simulink model "BLDC_speedcontrol_PWM"  (R2018a)
settings: Solver=ode45  StartTime=0.0  StopTime=2  FixedStep=Ts  MaxStep=.000001  RelTol=1e-3  EnableMultiTasking=on
InitFcn:
  | Power = 425;
  | 
  | R=.64;
  | L=1e-3;
  | J=.142e-3;
  | B=0;
  | Km=1.194;
  | Vdc=60;
  | 
  | Ts=1e-6;
  | P=16;
undefined symbols (not defined in the file): Ke, sigbuilder_block
libraries: powerlib x12, simulink x12, powerlib_meascontrol x8, dspsigops x4
settings Model: Creator=TELE  LastModifiedBy=TELE
settings SolverCC: ZeroCrossAlgorithm=Adaptive
settings DataIOCC: LimitDataPoints=on  SaveFormat=Array
settings OptimizationCC: LifeSpan=inf
settings DebuggingCC: UnderspecifiedInitializationDetection=Classic  MergeDetectMultiDrivingBlocksExec=none  MaxConsecutiveZCsMsg=none  SolverPrmCheckMsg=warning  StateNameClashWarn=warning  SFUnexpectedBacktrackingDiag=warning  SFNoUnconditionalDefaultTransitionDiag=warning  SFExecutionAtInitializationDiag=none
settings HardwareCC: ProdBitPerPointer=32  ProdBitPerSizeT=32  ProdBitPerPtrDiffT=32  ProdLargestAtomicFloat=None  ProdIntDivRoundTo=Undefined  ProdEndianess=Unspecified  ProdWordSize=32  ProdHWDeviceType=32-bit Generic
settings ModelReferenceCC: PropagateSignalLabelsOutOfModel=off
settings CodeAppCC: StateflowObjectComments=on
settings GRTTargetCC: TargetLangStandard=C89/C90 (ANSI)  GeneratePreprocessorConditionals=Disable all
settings ConfigComp: CovMetricSettings=dw  CovHtmlReporting=on  CovSaveCumulativeToWorkspaceVar=on  CovSaveSingleToWorkspaceVar=on  CovExternalEMLEnable=off
settings SimscapeCC: SimscapeNormalizeSystem=off

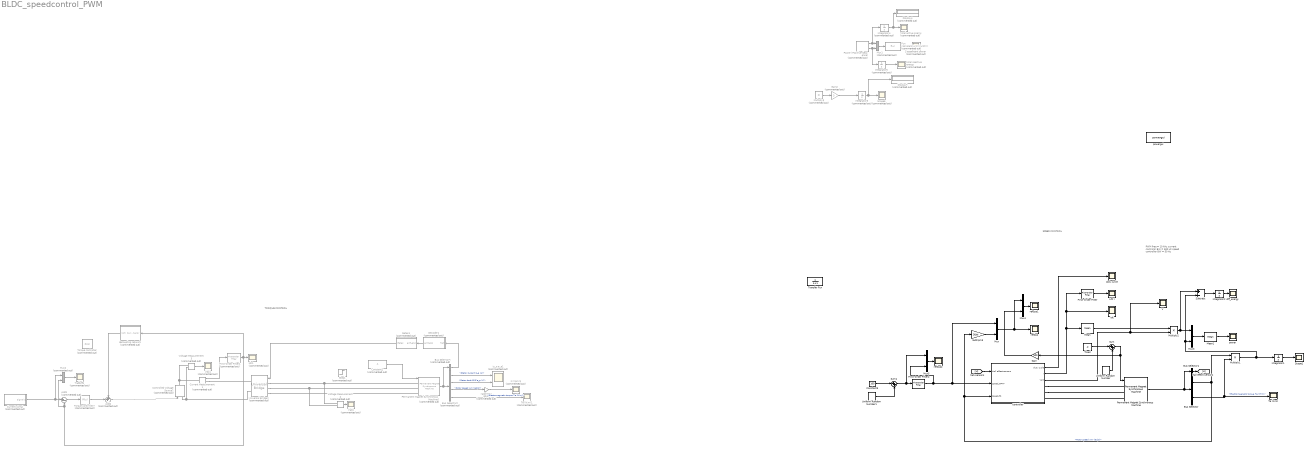
== system BLDC_speedcontrol_PWM ==
  note: SPEED CONTROL
  note: TORQUE CONTROL
  note: PWM freq = 10 kHz
      | current controler BW = 500 Hz
      | speed controller BW = 50 Hz
  Add1 : Sum  Commented=on  Inputs=|+-
  Add2 : Sum  Commented=on  Inputs=++|
  Bus Selector : BusSelector  OutputSignals=Rotor speed wm (rad/s),Electromagnetic torque Te (N*m)
  Bus Selector1 : BusSelector  OutputSignals=Hall effect signal h_a,Hall effect signal h_b,Hall effect signal h_c  OutputAsBus=on
  Bus Selector2 : BusSelector  Commented=on  OutputSignals=Stator current is_a (A),Stator back EMF e_a (V),Rotor speed wm (rad/s),Electromagnetic torque Te (N*m)
  Bus Selector3 : BusSelector  Commented=on  OutputSignals=Hall effect signal h_a,Hall effect signal h_b,Hall effect signal h_c  OutputAsBus=on
  Constant2 : Constant  Commented=on  Value=.1
  Constant3 : Constant  Value=100
  Controlled Voltage Source2 : powerlib/Electrical Sources/Controlled Voltage Source  Commented=on  Initialize=on  Source_Type=AC  Amplitude=500  Phase=0  Frequency=0  Measurements=None
  Current signal : Subsystem  Tag=STV Subsys  Commented=on  LoadFcn=sigbuilder_block('load');  StartFcn=sigbuilder_block('start');  StopFcn=sigbuilder_block('stop');  ClipboardFcn=sigbuilder_block('clipboard');  mask(Sigbuilder block){tuvar=[0:10]}
      mask help: Simulink:masks:SigbuilderBlock_MD
      mask init:
      | if ~strcmp(get_param(bdroot(gcbh),'SimulationStatus'),'stopped') tuvar = sigbuilder_block('maskInit'); end
      settings: CopyFcn=sigbuilder_block('copy');  DeleteFcn=sigbuilder_block('delete');  ModelCloseFcn=sigbuilder_block('modelClose');  PreSaveFcn=sigbuilder_block('preSave');  PauseFcn=sigbuilder_block('pause');  ContinueFcn=sigbuilder_block('continue');  NameChangeFcn=sigbuilder_block('namechange');  OpenFcn=sigbuilder_block('open',[437.25 180 550.5 395.25 ]);  CloseFcn=sigbuilder_block('close');
      mask Display: plot(0, 0, 100, 100,[2, 2, 32, 32, 2], [68, 8, 8, 68, 68],[32, 2], [38, 38], [32, 19, 2],[53, 60, 44], [32, 17, 17, 2],[16, 16, 31, 31]);txt = getActiveGroup(gcbh);text(2, 100, txt,'verticalAlignment', 'top');
  Current Measurement1 : powerlib/Measurements/Current Measurement  Commented=on  PhasorSimulation=off  OutputType=Complex  PSBequivalent=0
  Decoder1 : Subsystem  Commented=on
  Display3 : Display  Commented=on
  Display4 : Display  Commented=on
  Fcn : Fcn  Commented=on  Expr=cos(atan((u(1))/(u(2))))
  First-Order Filter : powerlib_meascontrol/Filters/First-Order Filter  FilterType=Lowpass  Tc=1e-3  Ts=0  Initialize=on  Vac_Init=[0, 0, 0]  Vdc_Init=0  PlotResponse=off  FreqRange="[0,  200,  1]"
      settings: SourceProductName=Simscape Power Systems
  First-Order Filter1 : powerlib_meascontrol/Filters/First-Order Filter  Commented=on  FilterType=Lowpass  Tc=10e-3  Ts=0  Initialize=on  Vac_Init=[0, 0, 60]  Vdc_Init=0  PlotResponse=off  FreqRange="[0,  200,  1]"
      settings: SourceProductName=Simscape Power Systems
  First-Order Filter2 : powerlib_meascontrol/Filters/First-Order Filter  FilterType=Lowpass  Tc=1/50  Ts=0  Initialize=on  Vac_Init=[0, 0, 0]  Vdc_Init=0  PlotResponse=off  FreqRange="[0,  200,  1]"
      settings: SourceProductName=Simscape Power Systems
  Gain : Gain  Gain=100
  Gain2 : Gain  Commented=on  Gain=3
  Gates1 : Subsystem  Commented=on
  "Idc " : Scope
  Idc1 : Scope  Commented=on
  Integrator1 : Integrator
  Integrator2 : Integrator
  Integrator3 : Integrator  Commented=on
  Integrator4 : Integrator  Commented=on
  Integrator5 : Integrator  Commented=on
  LPF I : Scope
  Mean : powerlib_meascontrol/Measurements/Mean  Freq=60  Vinit=0  Ts=0
  Mean1 : powerlib_meascontrol/Measurements/Mean  Freq=60  Vinit=0  Ts=0
  Multiply1 : Product
  Multiply2 : Product
  Multiply3 : Product  Commented=on
  Mux{,3..5} (4 alike) : Mux  Inputs=2
  Mux1 : Mux  Commented=on  Inputs=2
  Mux2 : Mux  Commented=on  Inputs=2
  N (rpm)1 : Scope  Commented=on
  Permanent Magnet Synchronous Machine : powerlib/Machines/Permanent Magnet Synchronous Machine  NbPhases=3  FluxDistribution=Trapezoidal  RotorType=Round  MechanicalLoad=Torque Tm  PresetModel=No  ShowDetailedParameters=on  MeasurementBus=off  Resistance=R  Inductance=L  dqInductances=[8.5e-3,8.5e-3]  La=L  MachineConstant=Torque Constant (N.m / A_peak)  Flux=0.037313  VoltageCst=125.0354  TorqueCst=Km  Flat=120  Mechanical=[J B P 0]  PolePairs=4  InitialConditions=[0,0, 0,0]  InitialConditions5ph=[0 0 0 0 0 0]  TsPowergui=0  TsBlock=-1  RefAngle=90 degrees behind phase A axis (modified Park)
      settings: SourceProductName=Simscape Power Systems
  Permanent Magnet Synchronous Machine1 : powerlib/Machines/Permanent Magnet Synchronous Machine  Commented=on  NbPhases=3  FluxDistribution=Trapezoidal  RotorType=Round  MechanicalLoad=Torque Tm  PresetModel=No  ShowDetailedParameters=on  MeasurementBus=off  Resistance=R  Inductance=L  dqInductances=[8.5e-3, 8.5e-3]  La=0.000835  MachineConstant=Torque Constant (N.m / A_peak)  Flux=0.00425  VoltageCst=7.1209  TorqueCst=Kt  Flat=120  Mechanical=[ J, B 8]  PolePairs=8  InitialConditions=[0,0, 0,0]  InitialConditions5ph=[0 0 0 0 0 0]  TsPowergui=0  TsBlock=-1  RefAngle=90 degrees behind phase A axis (modified Park)
      settings: SourceProductName=Simscape Power Systems
  Power (Positive-Sequence) : powerlib_meascontrol/Measurements/Power (Positive-Sequence)  Commented=on  Freq=60  Vinit=[0, 0]  Iinit=[0, 0]  Ts=0
      settings: SourceProductName=Simscape Power Systems  SourceProductBaseCode=PS
  S appereant power : Scope  Commented=on
  Scope1 : Scope
  Scope6 : Scope  Commented=on
  Step1 : Step  Commented=on  After=.1  SampleTime=0
  Subtract : Sum  Inputs=+-
  Sum : Sum  Inputs=|++
  Sum1 : Sum  Inputs=|++
  Te (N.m) : Scope
  Te (N.m)1 : Scope  Commented=on
  Tload : Constant  Value=.2
  Torque controller : simulink/Continuous/PID Controller  Commented=on  Controller=PI  TimeDomain=Continuous-time  SampleTime=-1  IntegratorMethod=Forward Euler  FilterMethod=Forward Euler  Form=Parallel  UseFilter=on  ControllerParametersSource=internal  P=2.12871841993777  I=6083.3305788616*.5  D=-0.000138058001454029  N=230.258625302705  InitialConditionSource=internal  InitialConditionForIntegrator=0  InitialConditionForFilter=0  ExternalReset=none  LimitOutput=off  UpperSaturationLimit=inf  LowerSaturationLimit=-inf  LinearizeAsGain=on  AntiWindupMode=none  Kb=1  TrackingMode=off  Kt=1  PParamMin=[]  PParamMax=[]  IParamMin=[]  IParamMax=[]  DParamMin=[]  DParamMax=[]  NParamMin=[]  NParamMax=[]  KbParamMin=[]  KbParamMax=[]  KtParamMin=[]  KtParamMax=[]  POutMin=[]  POutMax=[]  IOutMin=[]  IOutMax=[]  DOutMin=[]  DOutMax=[]  NOutMin=[]  NOutMax=[]  KbOutMin=[]  KbOutMax=[]  KtOutMin=[]  KtOutMax=[]  IntegratorOutMin=[]  IntegratorOutMax=[]  FilterOutMin=[]  FilterOutMax=[]  SumOutMin=[]  SumOutMax=[]  SumI1OutMin=[]  SumI1OutMax=[]  SumI2OutMin=[]  SumI2OutMax=[]  SumI3OutMin=[]  SumI3OutMax=[]  SumDOutMin=[]  SumDOutMax=[]  SaturationOutMin=[]  SaturationOutMax=[]  IntegratorContinuousStateAttributes=''  IntegratorStateMustResolveToSignalObject=off  IntegratorRTWStateStorageClass=Auto  FilterContinuousStateAttributes=''  FilterStateMustResolveToSignalObject=off  FilterRTWStateStorageClass=Auto  DifferentiatorICPrevScaledInput=0  DifferentiatorOutMin=[]  DifferentiatorOutMax=[]  FilterDiffOutCoefMin=[]  FilterDiffOutCoefMax=[]  SumDenOutMin=[]  SumDenOutMax=[]  SumNumOutMin=[]  SumNumOutMax=[]  ReciprocalOutMin=[]  ReciprocalOutMax=[]  DivideOutMin=[]  DivideOutMax=[]  TunerSelectOption=Transfer Function Based (PID Tuner App)
  Torque controller2 : simulink/Continuous/PID Controller  Commented=on  Controller=PI  TimeDomain=Continuous-time  SampleTime=-1  IntegratorMethod=Forward Euler  FilterMethod=Forward Euler  Form=Parallel  UseFilter=on  ControllerParametersSource=internal  P=7.77723774722096  I=2722.31111979485  D=-0.000138058001454029  N=230.258625302705  InitialConditionSource=internal  InitialConditionForIntegrator=0  InitialConditionForFilter=0  ExternalReset=none  LimitOutput=off  UpperSaturationLimit=inf  LowerSaturationLimit=-inf  LinearizeAsGain=on  AntiWindupMode=none  Kb=1  TrackingMode=off  Kt=1  PParamMin=[]  PParamMax=[]  IParamMin=[]  IParamMax=[]  DParamMin=[]  DParamMax=[]  NParamMin=[]  NParamMax=[]  KbParamMin=[]  KbParamMax=[]  KtParamMin=[]  KtParamMax=[]  POutMin=[]  POutMax=[]  IOutMin=[]  IOutMax=[]  DOutMin=[]  DOutMax=[]  NOutMin=[]  NOutMax=[]  KbOutMin=[]  KbOutMax=[]  KtOutMin=[]  KtOutMax=[]  IntegratorOutMin=[]  IntegratorOutMax=[]  FilterOutMin=[]  FilterOutMax=[]  SumOutMin=[]  SumOutMax=[]  SumI1OutMin=[]  SumI1OutMax=[]  SumI2OutMin=[]  SumI2OutMax=[]  SumI3OutMin=[]  SumI3OutMax=[]  SumDOutMin=[]  SumDOutMax=[]  SaturationOutMin=[]  SaturationOutMax=[]  IntegratorContinuousStateAttributes=''  IntegratorStateMustResolveToSignalObject=off  IntegratorRTWStateStorageClass=Auto  FilterContinuousStateAttributes=''  FilterStateMustResolveToSignalObject=off  FilterRTWStateStorageClass=Auto  DifferentiatorICPrevScaledInput=0  DifferentiatorOutMin=[]  DifferentiatorOutMax=[]  FilterDiffOutCoefMin=[]  FilterDiffOutCoefMax=[]  SumDenOutMin=[]  SumDenOutMax=[]  SumNumOutMin=[]  SumNumOutMax=[]  ReciprocalOutMin=[]  ReciprocalOutMax=[]  DivideOutMin=[]  DivideOutMax=[]  TunerSelectOption=Transfer Function Based (PID Tuner App)
  Transfer Fcn : TransferFcn  Denominator=[1 1]
  Tref&Tfb : Scope  Commented=on
  Uniform Random Number : UniformRandomNumber  Minimum=0  SampleTime=.1
  Uniform Random Number1 : UniformRandomNumber  Minimum=0  Maximum=200  SampleTime=1/100
  Universal Bridge1 : powerlib/Power Electronics/Universal Bridge  Commented=on  Arms=3  SnubberResistance=5000  SnubberCapacitance=1e-6  Device=MOSFET / Diodes  Ron=1e-3  Lon=0  ForwardVoltages="[  0  0  ]"  ForwardVoltage=0  GTOparameters=[ 10e-6 , 20e-6 ]  IGBTparameters=[ 1e-6 , 2e-6 ]  Measurements=None  Measurements_2=None  converterType=Rectifier
  V : Scope
  Vab1 : Scope  Commented=on
  Vdc1 : Scope  Commented=on
  Voltage Measurement2 : powerlib/Measurements/Voltage Measurement  Commented=on  PhasorSimulation=off  OutputType=Complex  PSBequivalent=0
  Voltage Measurement3 : powerlib/Measurements/Voltage Measurement  Commented=on  PhasorSimulation=off  OutputType=Complex  PSBequivalent=0
  controller : Subsystem
  decoupling network : Subsystem  Commented=on
  diff_energy : Scope
  duty cycle : Scope
  is_a e_a1 : Scope  Commented=on  NumInputPorts=2
  power : Scope
  powergui : powerlib/powergui  Priority=2  SimulationMode=Continuous  SampleTime=Ts  frequency=60  Iterations=50  frequencyindice=0  Pbase=100e6  ErrMax=1e-4  UnitsV=kV  UnitsW=MW  buscounter=0  FunctionMessages=off  echomessages=off  EnableUseOfTLC=off  CurrentSourceSwitches=off  DisableSnubberDevices=off  DisableRonSwitches=off  DisableVfSwitches=off  DisplayEquations=off  SolverType=Tustin  Interpol=off  ExternalGateDelay=off  methode=off  Ts=0  x0status=blocks  SPID=off  SwTol=0  HookPort=off  RestoreLinks=warning  ResistiveCurrentMeasurement=off  Frange=[0:2:500]  Ylog=off  Xlog=on  ShowGrid=off  save=off  variable=ZData  structure=0  ZoomFFT=on  StartTime=0.0  cycles=1  DisplayStyle=1  fundamental=60  FreqAxis=off  MaxFrequency=1000  frequencyindicesteady=1  RmsSteady=1  display=off
  rad2rpm1 : Gain  Commented=on  Gain=30/pi
  rad2rpm3 : Gain  Gain=30/pi
  ref&sp : Scope
  ref&sp1 : Scope
  ref&sp2 : Scope
  total active energy : Scope  Commented=on
  total reactive energy : Scope  Commented=on
  wires:
  Permanent Magnet Synchronous Machine/1 -> Bus Selector1/1, Bus Selector/1
  Bus Selector1/1 -> [H]
  Bus Selector/1 -> Multiply1/1, rad2rpm3/1, controller/3(speed_fb)  "<Rotor speed wm (rad/s)>"
  Bus Selector/2 -> Multiply1/2, Te (N.m)/1  "<Electromagnetic torque Te (N*m)>"
  Gates1/1(Gates) -> Universal Bridge1/1
  Decoder1/1(emf_abc) -> Gates1/1("emf_abc ")
  rad2rpm1/1 -> N (rpm)1/1
  Voltage Measurement2/1 -> Vab1/1
  Voltage Measurement3/1 -> Vdc1/1
  Bus Selector2/1 -> is_a e_a1/1  "<Stator current is_a (A)>"
  Permanent Magnet Synchronous Machine1/1 -> Bus Selector2/1, Bus Selector3/1
  Bus Selector3/1 -> Decoder1/1("Hall ")
  Bus Selector2/2 -> is_a e_a1/2  "<Stator back EMF e_a (V)>"
  Bus Selector2/3 -> rad2rpm1/1  "<Rotor speed wm (rad/s)>"
  Bus Selector2/4 -> Te (N.m)1/1  "<Electromagnetic torque Te (N*m)>"
  Current Measurement1/1 -> First-Order Filter1/1
  Add1/1 -> Torque controller2/1
  Mux2/1 -> Tref&Tfb/1
  First-Order Filter1/1 -> decoupling network/1(Current error), Mux2/2, Add1/2, Idc1/1
  Current signal/1(Signal 1) -> Mux2/1, Add1/1
  Constant2/1 -> Permanent Magnet Synchronous Machine1/1
  Torque controller2/1 -> Add2/2
  Add2/1 -> Controlled Voltage Source2/1
  decoupling network/1(Volt) -> Add2/1
  [H] -> controller/1(Hall effect sensors)
  controller/1(duty cycle) -> duty cycle/1
  Integrator1/1 -> Scope1/1
  Mux/1 -> ref&sp/1, Mux4/1
  rad2rpm3/1 -> Mux/2
  Gain2/1 -> Integrator3/1
  Integrator3/1 -> Display3/1, Scope6/1
  Multiply3/1 -> Gain2/1
  Integrator5/1 -> total reactive energy/1
  Power (Positive-Sequence)/1 -> Integrator4/1, Mux1/1
  Mux1/1 -> Fcn/1
  ? -> Power (Positive-Sequence)/2
  Integrator4/1 -> Display4/1, total active energy/1
  Fcn/1 -> S appereant power/1
  Power (Positive-Sequence)/2 -> Integrator5/1, Mux1/2
  ? -> Power (Positive-Sequence)/1
  Tload/1 -> Sum/1
  controller/2(I) -> First-Order Filter/1, "Idc "/1, Mean/1
  First-Order Filter/1 -> LPF I/1
  Subtract/1 -> Integrator2/1
  Mean/1 -> Multiply2/1
  controller/3(Volt) -> V/1, Multiply2/2
  Mux3/1 -> Mean1/1
  Multiply2/1 -> Subtract/1, Mux3/1
  Multiply1/1 -> Subtract/2, Mux3/2, Integrator1/1
  Integrator2/1 -> diff_energy/1
  Uniform Random Number/1 -> Sum/2
  Mux4/1 -> ref&sp1/1
  Sum/1 -> Permanent Magnet Synchronous Machine/1, Gain/1
  Gain/1 -> Mux4/2
  Mean1/1 -> power/1
  Sum1/1 -> First-Order Filter2/1, Mux5/1
  Mux5/1 -> ref&sp2/1
  Constant3/1 -> Sum1/1
  Uniform Random Number1/1 -> Sum1/2
  First-Order Filter2/1 -> Mux5/2, Mux/1, controller/2(speed_RPM*)
  connections:
  Universal Bridge1/LConn1 -- Voltage Measurement2/LConn1 -- Permanent Magnet Synchronous Machine1/LConn1
  Universal Bridge1/LConn2 -- Voltage Measurement2/LConn2 -- Permanent Magnet Synchronous Machine1/LConn2
  Controlled Voltage Source2/RConn1 -- Current Measurement1/LConn1 -- Voltage Measurement3/LConn1
  Controlled Voltage Source2/LConn1 -- Voltage Measurement3/LConn2 -- Universal Bridge1/RConn2
  Universal Bridge1/LConn3 -- Permanent Magnet Synchronous Machine1/LConn3
  Current Measurement1/RConn1 -- Universal Bridge1/RConn1
  Permanent Magnet Synchronous Machine/LConn3 -- controller/RConn3
  controller/RConn2 -- Permanent Magnet Synchronous Machine/LConn2
  controller/RConn1 -- Permanent Magnet Synchronous Machine/LConn1

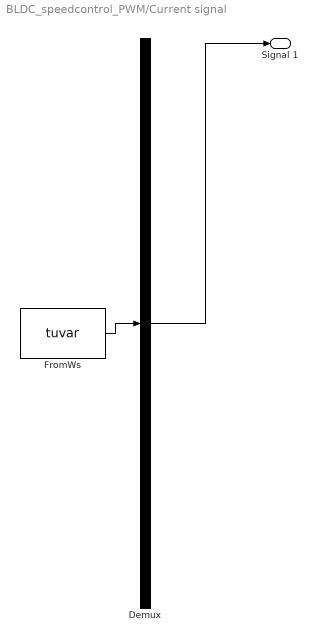
== system BLDC_speedcontrol_PWM/Current signal ==
  Demux : Demux  Tag=STV Demux  Outputs=1
  FromWs : FromWorkspace  Tag=STV FromWs  VariableName=tuvar  SampleTime=0
      SigBuilderData=|
      | common.afterFinalStr = 'Extrapolate'
      | common.sampleTime = 0
      | dataSet.timeRange = [0 10]
      | dataSet.name = 'Group 1'
      | sbobj.Groups.Name = 'Group 1'
      | sbobj.Groups.Signals.Name = 'Signal 1'
      | sbobj.Groups.Signals.XData = [0 0.22 0.22 2 2 10]
      | sbobj.Groups.Signals.YData = [0 0 2 2 0 0]
  Signal 1 : Outport  Tag=STV Outport
  wires:
  FromWs/1 -> Demux/1
  Demux/1 -> Signal 1/1

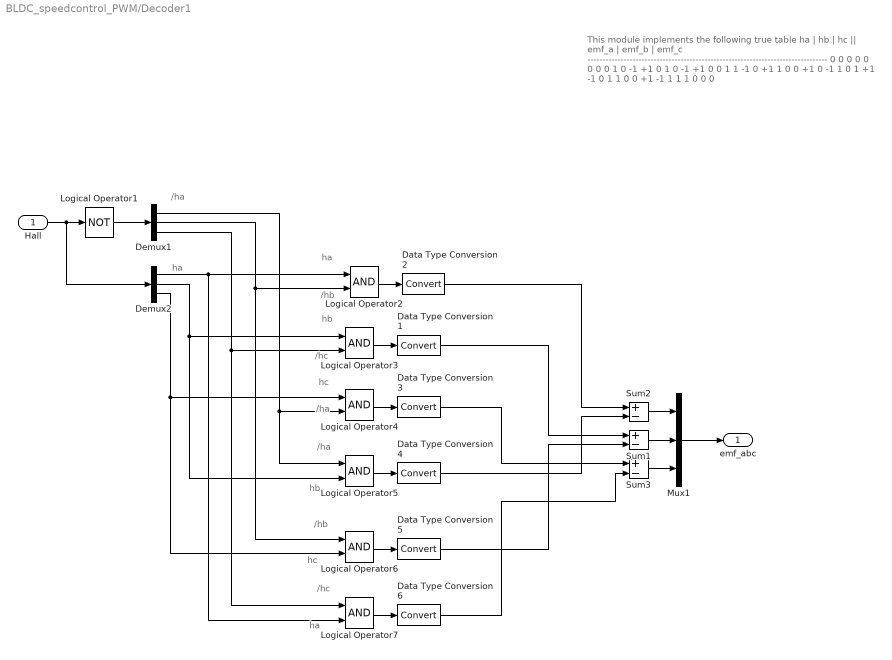
== system BLDC_speedcontrol_PWM/Decoder1 ==
  note: /ha
  note: ha
  note: ha
  note: /hb
  note: hb
  note: /hc
  note: hc
  note: /ha
  note: /ha
  note: hb
  note: /hb
  note: hc
  note: /hc
  note: ha
  note: This module implements the following true table
      |
      |    ha   |   hb   |   hc   ||   emf_a   |   emf_b   |   emf_c
      |     --------------------------------------------------------------------------------
      | 0          0         0          0               0               0
      | 0          0         1          0               -1              +1
      | 0          1         0          -1              +1                0
      | 0          1         1          -1               0               +1
      | 1          0         0         +1               0               -1
      | 1          0         1         +1              -1                0
      | 1          1         0          0              +1               -1
      | 1          1         1          0               0                0
  "Hall " : Inport
  Data Type Conversion{1..6} (6 alike) : DataTypeConversion
  Demux1 : Demux  Outputs=3
  Demux2 : Demux  Outputs=3
  Logical Operator1 : Logic  Operator=NOT  AllPortsSameDT=off  OutDataTypeStr=boolean
  Logical Operator{2..7} (6 alike) : Logic  AllPortsSameDT=off  OutDataTypeStr=boolean
  Mux1 : Mux  Inputs=3
  Sum1 : Sum  Inputs=+-  OutDataTypeStr=double
  Sum2 : Sum  Inputs=+-  OutDataTypeStr=double
  Sum3 : Sum  Inputs=+-  OutDataTypeStr=double
  emf_abc : Outport
  wires:
  "Hall "/1 -> Logical Operator1/1, Demux2/1
  Logical Operator1/1 -> Demux1/1
  Demux2/3 -> Logical Operator4/1, Logical Operator6/2
  Demux2/2 -> Logical Operator3/1, Logical Operator5/2
  Demux2/1 -> Logical Operator2/1, Logical Operator7/2
  Demux1/3 -> Logical Operator3/2, Logical Operator7/1
  Demux1/2 -> Logical Operator2/2, Logical Operator6/1
  Demux1/1 -> Logical Operator4/2, Logical Operator5/1
  Logical Operator2/1 -> Data Type Conversion2/1
  Sum2/1 -> Mux1/1
  Sum1/1 -> Mux1/2
  Sum3/1 -> Mux1/3
  Mux1/1 -> emf_abc/1
  Logical Operator3/1 -> Data Type Conversion1/1
  Logical Operator4/1 -> Data Type Conversion3/1
  Logical Operator5/1 -> Data Type Conversion4/1
  Logical Operator6/1 -> Data Type Conversion5/1
  Logical Operator7/1 -> Data Type Conversion6/1
  Data Type Conversion2/1 -> Sum2/1
  Data Type Conversion4/1 -> Sum2/2
  Data Type Conversion1/1 -> Sum1/1
  Data Type Conversion5/1 -> Sum1/2
  Data Type Conversion3/1 -> Sum3/1
  Data Type Conversion6/1 -> Sum3/2

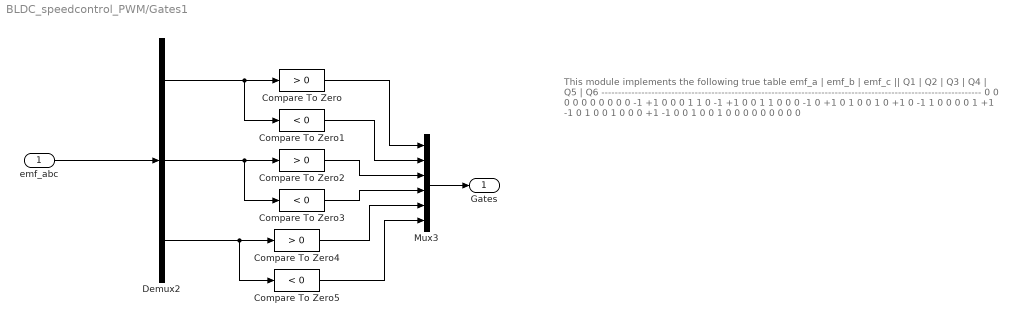
== system BLDC_speedcontrol_PWM/Gates1 ==
  note: This module implements the following true table
      |
      |    emf_a   |   emf_b   |   emf_c   ||   Q1   |   Q2   |   Q3   |   Q4   |   Q5   |   Q6
      |     ------------------------------------------------------------------------------------------------------------------
      |       0              0                0            0          0          0           0        0        0
      |       0               -1              +1          0          0          0           1        1        0
      |     -1              +1                0          0          1          1           0        0        0
      |     -1               0               +1          0          1         0           0        1        0
      |    +1               0                -1          1          0          0           0        0        1
      |    +1              -1                0           1          0          0           1        0        0
      |      0              +1               -1           0          0          1           0        0        1
      |     0              0                0             0          0          0           0        0        0
  "emf_abc " : Inport
  Compare To Zero : simulink/Logic and Bit Operations/Compare To Zero  relop=>  OutDataTypeStr=boolean  ZeroCross=off
  Compare To Zero1 : simulink/Logic and Bit Operations/Compare To Zero  relop=<  OutDataTypeStr=boolean  ZeroCross=off
  Compare To Zero2 : simulink/Logic and Bit Operations/Compare To Zero  relop=>  OutDataTypeStr=boolean  ZeroCross=off
  Compare To Zero3 : simulink/Logic and Bit Operations/Compare To Zero  relop=<  OutDataTypeStr=boolean  ZeroCross=off
  Compare To Zero4 : simulink/Logic and Bit Operations/Compare To Zero  relop=>  OutDataTypeStr=boolean  ZeroCross=off
  Compare To Zero5 : simulink/Logic and Bit Operations/Compare To Zero  relop=<  OutDataTypeStr=boolean  ZeroCross=off
  Demux2 : Demux  Outputs=3
  Mux3 : Mux  Inputs=6
  Gates : Outport
  wires:
  "emf_abc "/1 -> Demux2/1
  Mux3/1 -> Gates/1
  Demux2/1 -> Compare To Zero/1, Compare To Zero1/1
  Demux2/2 -> Compare To Zero2/1, Compare To Zero3/1
  Demux2/3 -> Compare To Zero4/1, Compare To Zero5/1
  Compare To Zero/1 -> Mux3/1
  Compare To Zero1/1 -> Mux3/2
  Compare To Zero2/1 -> Mux3/3
  Compare To Zero3/1 -> Mux3/4
  Compare To Zero4/1 -> Mux3/5
  Compare To Zero5/1 -> Mux3/6

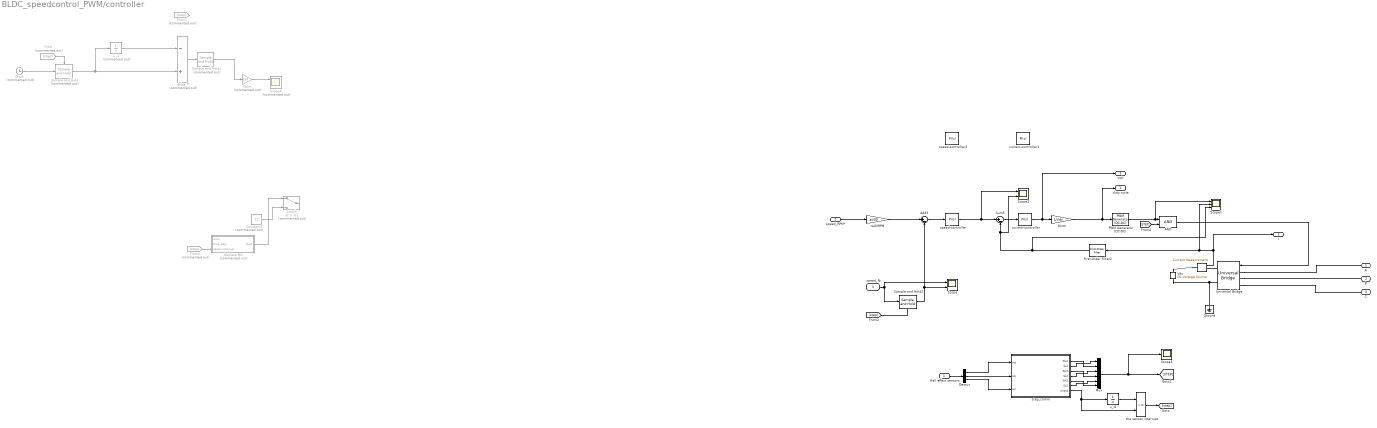
== system BLDC_speedcontrol_PWM/controller ==
  Hall effect sensors : Inport
  speed_RPM* : Inport  Port=2
  speed_fb : Inport  Port=3
  ' : powerlib/Measurements/Current Measurement  PhasorSimulation=off  OutputType=Complex  PSBequivalent=0
  AND : Logic  AllPortsSameDT=off  OutDataTypeStr=boolean
  Add3 : Sum  Inputs=|+-
  Clock : Clock  Commented=on
  Constant1 : Constant  Commented=on  Value=12
  Demux : Demux  Outputs=3
  First-Order Filter2 : powerlib_meascontrol/Filters/First-Order Filter  FilterType=Lowpass  Tc=1e-3  Ts=0  Initialize=on  Vac_Init=[0, 0, 0]  Vdc_Init=0  PlotResponse=off  FreqRange="[0,  200,  1]"
      settings: SourceProductName=Simscape Power Systems
  From : From  Commented=on  GotoTag=step
  From1 : From  Commented=on  GotoTag=step
  From3 : From  Commented=on  GotoTag=step
  Gain : Gain  Commented=on  Gain=1e3
  Ground : powerlib/Elements/Ground  LConnTagsString=a
  Mux : Mux  Inputs=6
  Norm : Gain  Gain=1/Vdc
  PWM Generator (DC-DC) : powerlib_meascontrol/Pulse & Signal Generators/PWM Generator (DC-DC)  Fsw=20e3  Ts=0
  Sample and Hold : dspsigops/Sample and Hold  Commented=on  trig=Rising edge  initCond=0  latchinput=off
  Sample and Hold1 : dspsigops/Sample and Hold  Commented=on  trig=Rising edge  initCond=0  latchinput=off
  Sample and Hold2 : dspsigops/Sample and Hold  trig=Rising edge  initCond=0  latchinput=off
  Scope : Scope  NumInputPorts=2
  Scope1 : Scope  NumInputPorts=3
  Scope2 : Scope  NumInputPorts=2
  Scope4 : Scope  Commented=on  NumInputPorts=2
  Scope5 : Scope
  Sum5 : Sum  Inputs=|+-
  Switch : Switch  Commented=on  Criteria=u2 > Threshold  Threshold=.01
  Universal Bridge : powerlib/Power Electronics/Universal Bridge  Arms=3  SnubberResistance=5000  SnubberCapacitance=1e-6  Device=MOSFET / Diodes  Ron=1e-3  Lon=0  ForwardVoltages="[  0  0  ]"  ForwardVoltage=0  GTOparameters=[ 10e-6 , 20e-6 ]  IGBTparameters=[ 1e-6 , 2e-6 ]  Measurements=None  Measurements_2=None  converterType=Rectifier
  Vdc : powerlib/Electrical Sources/DC Voltage Source  Amplitude=Vdc  Measurements=None
  current-controller : simulink/Continuous/PID Controller  Controller=PI  TimeDomain=Continuous-time  SampleTime=-1  IntegratorMethod=Forward Euler  FilterMethod=Forward Euler  Form=Parallel  UseFilter=on  ControllerParametersSource=internal  P=.01  I=479.896371550439  D=-0.000138058001454029  N=230.258625302705  InitialConditionSource=internal  InitialConditionForIntegrator=0  InitialConditionForFilter=0  ExternalReset=none  LimitOutput=on  UpperSaturationLimit=Vdc  LowerSaturationLimit=0  LinearizeAsGain=on  AntiWindupMode=clamping  Kb=1  TrackingMode=off  Kt=1  PParamMin=[]  PParamMax=[]  IParamMin=[]  IParamMax=[]  DParamMin=[]  DParamMax=[]  NParamMin=[]  NParamMax=[]  KbParamMin=[]  KbParamMax=[]  KtParamMin=[]  KtParamMax=[]  POutMin=[]  POutMax=[]  IOutMin=[]  IOutMax=[]  DOutMin=[]  DOutMax=[]  NOutMin=[]  NOutMax=[]  KbOutMin=[]  KbOutMax=[]  KtOutMin=[]  KtOutMax=[]  IntegratorOutMin=[]  IntegratorOutMax=[]  FilterOutMin=[]  FilterOutMax=[]  SumOutMin=[]  SumOutMax=[]  SumI1OutMin=[]  SumI1OutMax=[]  SumI2OutMin=[]  SumI2OutMax=[]  SumI3OutMin=[]  SumI3OutMax=[]  SumDOutMin=[]  SumDOutMax=[]  SaturationOutMin=[]  SaturationOutMax=[]  IntegratorContinuousStateAttributes=''  IntegratorStateMustResolveToSignalObject=off  IntegratorRTWStateStorageClass=Auto  FilterContinuousStateAttributes=''  FilterStateMustResolveToSignalObject=off  FilterRTWStateStorageClass=Auto  DifferentiatorICPrevScaledInput=0  DifferentiatorOutMin=[]  DifferentiatorOutMax=[]  FilterDiffOutCoefMin=[]  FilterDiffOutCoefMax=[]  SumDenOutMin=[]  SumDenOutMax=[]  SumNumOutMin=[]  SumNumOutMax=[]  ReciprocalOutMin=[]  ReciprocalOutMax=[]  DivideOutMin=[]  DivideOutMax=[]  TunerSelectOption=Transfer Function Based (PID Tuner App)
  current-controller1 : simulink/Continuous/PID Controller  Controller=PI  TimeDomain=Discrete-time  SampleTime=.0002  IntegratorMethod=Trapezoidal  FilterMethod=Forward Euler  Form=Parallel  UseFilter=on  ControllerParametersSource=internal  P=0.228414146935332  I=376.292717854929  D=-0.000138058001454029  N=230.258625302705  InitialConditionSource=internal  InitialConditionForIntegrator=0  InitialConditionForFilter=0  ExternalReset=none  LimitOutput=on  UpperSaturationLimit=Vdc  LowerSaturationLimit=0  LinearizeAsGain=on  AntiWindupMode=clamping  Kb=1  TrackingMode=off  Kt=1  PParamMin=[]  PParamMax=[]  IParamMin=[]  IParamMax=[]  DParamMin=[]  DParamMax=[]  NParamMin=[]  NParamMax=[]  KbParamMin=[]  KbParamMax=[]  KtParamMin=[]  KtParamMax=[]  POutMin=[]  POutMax=[]  IOutMin=[]  IOutMax=[]  DOutMin=[]  DOutMax=[]  NOutMin=[]  NOutMax=[]  KbOutMin=[]  KbOutMax=[]  KtOutMin=[]  KtOutMax=[]  IntegratorOutMin=[]  IntegratorOutMax=[]  FilterOutMin=[]  FilterOutMax=[]  SumOutMin=[]  SumOutMax=[]  SumI1OutMin=[]  SumI1OutMax=[]  SumI2OutMin=[]  SumI2OutMax=[]  SumI3OutMin=[]  SumI3OutMax=[]  SumDOutMin=[]  SumDOutMax=[]  SaturationOutMin=[]  SaturationOutMax=[]  IntegratorContinuousStateAttributes=''  IntegratorStateMustResolveToSignalObject=off  IntegratorRTWStateStorageClass=Auto  FilterContinuousStateAttributes=''  FilterStateMustResolveToSignalObject=off  FilterRTWStateStorageClass=Auto  DifferentiatorICPrevScaledInput=0  DifferentiatorOutMin=[]  DifferentiatorOutMax=[]  FilterDiffOutCoefMin=[]  FilterDiffOutCoefMax=[]  SumDenOutMin=[]  SumDenOutMax=[]  SumNumOutMin=[]  SumNumOutMax=[]  ReciprocalOutMin=[]  ReciprocalOutMax=[]  DivideOutMin=[]  DivideOutMax=[]  TunerSelectOption=Transfer Function Based (PID Tuner App)
  delta_T : Sum  Commented=on  Inputs=-+
  discrete PID : Subsystem  Commented=on
  rad2RPM : Gain  Gain=pi/30
  speed-controller : simulink/Continuous/PID Controller  Controller=PI  TimeDomain=Continuous-time  SampleTime=-1  IntegratorMethod=Forward Euler  FilterMethod=Forward Euler  Form=Parallel  UseFilter=on  ControllerParametersSource=internal  P=0.185814513304236  I=4.94881180882956  D=-0.000138058001454029  N=230.258625302705  InitialConditionSource=internal  InitialConditionForIntegrator=0  InitialConditionForFilter=0  ExternalReset=none  LimitOutput=on  UpperSaturationLimit=Vdc  LowerSaturationLimit=0  LinearizeAsGain=on  AntiWindupMode=clamping  Kb=1  TrackingMode=off  Kt=1  PParamMin=[]  PParamMax=[]  IParamMin=[]  IParamMax=[]  DParamMin=[]  DParamMax=[]  NParamMin=[]  NParamMax=[]  KbParamMin=[]  KbParamMax=[]  KtParamMin=[]  KtParamMax=[]  POutMin=[]  POutMax=[]  IOutMin=[]  IOutMax=[]  DOutMin=[]  DOutMax=[]  NOutMin=[]  NOutMax=[]  KbOutMin=[]  KbOutMax=[]  KtOutMin=[]  KtOutMax=[]  IntegratorOutMin=[]  IntegratorOutMax=[]  FilterOutMin=[]  FilterOutMax=[]  SumOutMin=[]  SumOutMax=[]  SumI1OutMin=[]  SumI1OutMax=[]  SumI2OutMin=[]  SumI2OutMax=[]  SumI3OutMin=[]  SumI3OutMax=[]  SumDOutMin=[]  SumDOutMax=[]  SaturationOutMin=[]  SaturationOutMax=[]  IntegratorContinuousStateAttributes=''  IntegratorStateMustResolveToSignalObject=off  IntegratorRTWStateStorageClass=Auto  FilterContinuousStateAttributes=''  FilterStateMustResolveToSignalObject=off  FilterRTWStateStorageClass=Auto  DifferentiatorICPrevScaledInput=0  DifferentiatorOutMin=[]  DifferentiatorOutMax=[]  FilterDiffOutCoefMin=[]  FilterDiffOutCoefMax=[]  SumDenOutMin=[]  SumDenOutMax=[]  SumNumOutMin=[]  SumNumOutMax=[]  ReciprocalOutMin=[]  ReciprocalOutMax=[]  DivideOutMin=[]  DivideOutMax=[]  TunerSelectOption=Transfer Function Based (PID Tuner App)
  speed-controller2 : simulink/Continuous/PID Controller  Controller=PI  TimeDomain=Discrete-time  SampleTime=.0002  IntegratorMethod=Trapezoidal  FilterMethod=Forward Euler  Form=Parallel  UseFilter=on  ControllerParametersSource=internal  P=0.127599674617565  I=1.78394081781165  D=-0.000138058001454029  N=230.258625302705  InitialConditionSource=internal  InitialConditionForIntegrator=0  InitialConditionForFilter=0  ExternalReset=none  LimitOutput=on  UpperSaturationLimit=Vdc  LowerSaturationLimit=0  LinearizeAsGain=on  AntiWindupMode=clamping  Kb=1  TrackingMode=off  Kt=1  PParamMin=[]  PParamMax=[]  IParamMin=[]  IParamMax=[]  DParamMin=[]  DParamMax=[]  NParamMin=[]  NParamMax=[]  KbParamMin=[]  KbParamMax=[]  KtParamMin=[]  KtParamMax=[]  POutMin=[]  POutMax=[]  IOutMin=[]  IOutMax=[]  DOutMin=[]  DOutMax=[]  NOutMin=[]  NOutMax=[]  KbOutMin=[]  KbOutMax=[]  KtOutMin=[]  KtOutMax=[]  IntegratorOutMin=[]  IntegratorOutMax=[]  FilterOutMin=[]  FilterOutMax=[]  SumOutMin=[]  SumOutMax=[]  SumI1OutMin=[]  SumI1OutMax=[]  SumI2OutMin=[]  SumI2OutMax=[]  SumI3OutMin=[]  SumI3OutMax=[]  SumDOutMin=[]  SumDOutMax=[]  SaturationOutMin=[]  SaturationOutMax=[]  IntegratorContinuousStateAttributes=''  IntegratorStateMustResolveToSignalObject=off  IntegratorRTWStateStorageClass=Auto  FilterContinuousStateAttributes=''  FilterStateMustResolveToSignalObject=off  FilterRTWStateStorageClass=Auto  DifferentiatorICPrevScaledInput=0  DifferentiatorOutMin=[]  DifferentiatorOutMax=[]  FilterDiffOutCoefMin=[]  FilterDiffOutCoefMax=[]  SumDenOutMin=[]  SumDenOutMax=[]  SumNumOutMin=[]  SumNumOutMax=[]  ReciprocalOutMin=[]  ReciprocalOutMax=[]  DivideOutMin=[]  DivideOutMax=[]  TunerSelectOption=Transfer Function Based (PID Tuner App)
  step_comm : MATLAB Function  TreatAsAtomicUnit=on
  the sensor interrupt : RelationalOperator  Operator=~=  OutDataTypeStr=boolean  RndMeth=Simplest
  u_-1 : UnitDelay  Commented=on  SampleTime=-1
  u_-6 : UnitDelay  SampleTime=-1
  A : PMIOPort  Side=Right
  B : PMIOPort  Port=2  Side=Right
  C : PMIOPort  Port=3  Side=Right
  duty cycle : Outport
  I : Outport  Port=2
  Volt : Outport  Port=3
  wires:
  AND/1 -> Universal Bridge/1
  '/1 -> Scope1/2, First-Order Filter2/1, I/1
  rad2RPM/1 -> Add3/1
  speed_RPM*/1 -> rad2RPM/1
  Hall effect sensors/1 -> Demux/1
  step_comm/5(SH3) -> Mux/6
  step_comm/6(SL3) -> Mux/5
  step_comm/1(SH1) -> Mux/2
  step_comm/2(SL1) -> Mux/1
  step_comm/4(SL2) -> Mux/3
  step_comm/3(SH2) -> Mux/4
  PWM Generator (DC-DC)/1 -> Scope1/1, AND/1
  Mux/1 -> [STEP], Scope5/1
  Clock/1 -> Sample and Hold/1
  u_-6/1 -> the sensor interrupt/1
  the sensor interrupt/1 -> [step]
  Sample and Hold/1 -> u_-1/1, delta_T/2
  Sample and Hold1/1 -> Gain/1
  From/1 -> Sample and Hold/Trigger
  u_-1/1 -> delta_T/1
  delta_T/1 -> Sample and Hold1/1
  step_comm/7(phase) -> the sensor interrupt/2, u_-6/1
  Gain/1 -> Scope4/1
  discrete PID/1(Out1) -> Switch/1
  From3/1 -> discrete PID/3(sensor interrupt)
  Constant1/1 -> Switch/3
  speed_fb/1 -> Sample and Hold2/1, Scope/1
  Add3/1 -> speed-controller/1
  [step] -> Sample and Hold2/Trigger
  Demux/2 -> step_comm/2(Hb)
  Demux/1 -> step_comm/1(Ha)
  Demux/3 -> step_comm/3(Hc)
  [STEP] -> AND/2
  Sum5/1 -> current-controller/1
  speed-controller/1 -> Scope2/1, Sum5/1
  Norm/1 -> duty cycle/1, PWM Generator (DC-DC)/1
  First-Order Filter2/1 -> Scope1/3, Scope2/2, Sum5/2
  current-controller/1 -> Volt/1, Norm/1
  Sample and Hold2/1 -> Scope/2, Add3/2
  connections:
  Universal Bridge/LConn1 -- A/RConn1
  Universal Bridge/LConn3 -- C/RConn1
  Universal Bridge/RConn1 -- '/RConn1
  Vdc/LConn1 -- Ground/LConn1 -- Universal Bridge/RConn2
  Universal Bridge/LConn2 -- B/RConn1
  '/LConn1 -- Vdc/RConn1

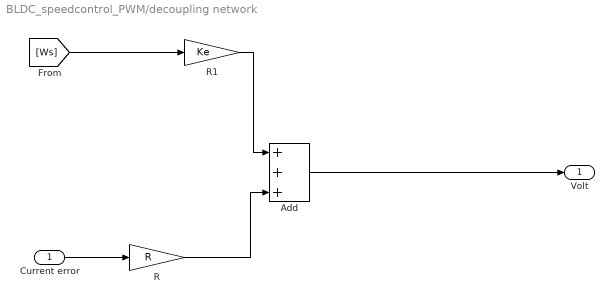
== system BLDC_speedcontrol_PWM/decoupling network ==
  Current error : Inport
  Add : Sum  Inputs=+++
  R : Gain  Gain=R
  R1 : Gain  Gain=Ke
  Volt : Outport
  wires:
  Current error/1 -> R/1
  R1/1 -> Add/1
  [Ws] -> R1/1
  Add/1 -> Volt/1
  R/1 -> Add/3

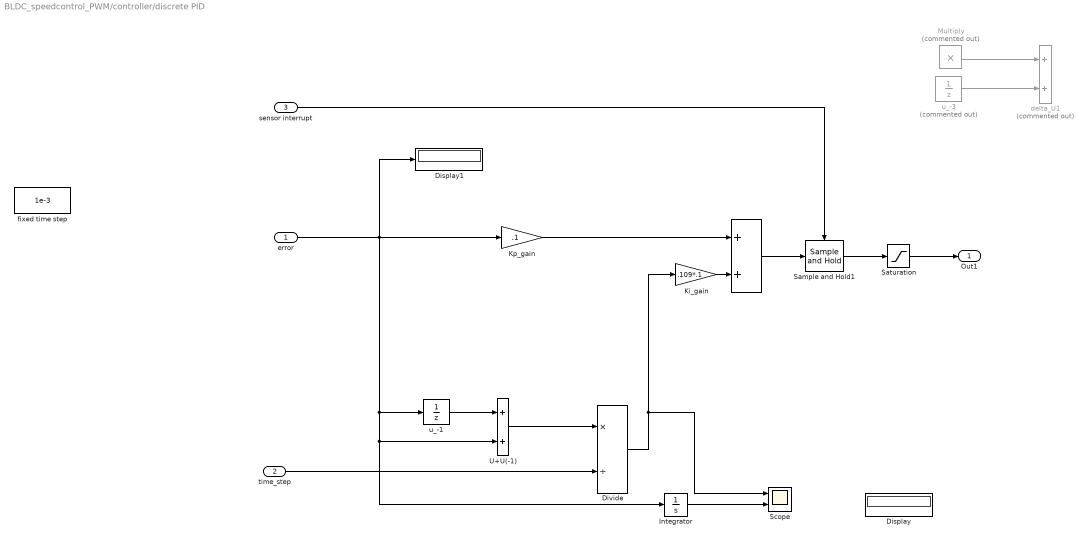
== system BLDC_speedcontrol_PWM/controller/discrete PID ==
  error : Inport
  time_step : Inport  Port=2
  sensor interrupt : Inport  Port=3
  " " : Sum  Inputs=2
  Display : Display
  Display1 : Display
  Divide : Product  Inputs=*/
  Integrator : Integrator
  Ki_gain : Gain  Gain=.109*.1
  "Kp_gain " : Gain  Gain=.1
  Multiply : Product  Commented=on
  Sample and Hold1 : dspsigops/Sample and Hold  trig=Rising edge  initCond=0  latchinput=off
  Saturation : Saturate  UpperLimit=Vdc  LowerLimit=0
  Scope : Scope  NumInputPorts=2
  U+U(-1) : Sum
  delta_U1 : Sum  Commented=on
  fixed time step : Constant  Value=1e-3
  u_-1 : UnitDelay  SampleTime=-1
  u_-3 : UnitDelay  Commented=on  SampleTime=-1
  Out1 : Outport
  wires:
  error/1 -> Integrator/1, U+U(-1)/2, u_-1/1, Display1/1, "Kp_gain "/1
  "Kp_gain "/1 -> " "/1
  u_-1/1 -> U+U(-1)/1
  Ki_gain/1 -> " "/2
  U+U(-1)/1 -> Divide/1
  time_step/1 -> Divide/2
  Multiply/1 -> delta_U1/1
  u_-3/1 -> delta_U1/2
  Divide/1 -> Scope/1, Ki_gain/1
  " "/1 -> Sample and Hold1/1
  Saturation/1 -> Out1/1
  Integrator/1 -> Scope/2
  Sample and Hold1/1 -> Saturation/1
  sensor interrupt/1 -> Sample and Hold1/Trigger

== matlab function BLDC_speedcontrol_PWM/controller/step_comm ==
  data: Ha input; SH1 output; Hb input; Hc input; SL1 output; SH2 output; SL2 output; SH3 output; SL3 output; phase output
function [SH1,SL1,SH2,SL2,SH3,SL3,phase]= fcn(Ha,Hb,Hc)

if ( (Ha==1) && (Hb==0) && (Hc==0) )  
    SL1 = 1;
    SH1 = 0;
    SL2 = 0;
    SH2 = 0;
    SL3 = 0;
    SH3 = 1;  
    phase=6;
elseif ( (Ha==0) && (Hb==1) && (Hc==0) )   
    SL1 = 0;
    SH1 = 1;
    SL2 = 1;
    SH2 = 0;
    SL3 = 0;
    SH3 = 0;  
    phase=4;
elseif ( (Ha==1) && (Hb==1) && (Hc==0) )   
    SL1 = 0;
    SH1 = 0;
    SL2 = 1;
    SH2 = 0;
    SL3 = 0;
    SH3 = 1;  
    phase=5;
elseif ( (Ha==0) && (Hb==0) && (Hc==1) )   
    SL1 = 0;
    SH1 = 0;
    SL2 = 0;
    SH2 = 1;
    SL3 = 1;
    SH3 = 0;  
    phase=2;
elseif ( (Ha==1) && (Hb==0) && (Hc==1) )   
    SL1 = 1;
    SH1 = 0;
    SL2 = 0;
    SH2 = 1;
    SL3 = 0;
    SH3 = 0;  
    phase=1;
elseif ( (Ha==0) && (Hb==1) && (Hc==1) )   
    SL1 = 0;
    SH1 = 1;
    SL2 = 0;
    SH2 = 0;
    SL3 = 1;
    SH3 = 0;  
    phase=3;
else
    SL1 = 0;
    SH1 = 0;
    SL2 = 0;
    SH2 = 0;
    SL3 = 0;
    SH3 = 0;  
    phase=0;
end
